simulink model "inverter"  (Simulink 8.4)
settings: Solver=ode23tb  StartTime=0.0  StopTime=0.1  MaxStep=.00001  RelTol=1e-3
libraries: powerlib x25, simulink x1
settings Model: Creator=jagadeeswari  LastModifiedBy=SELVA
settings SolverCC: InitialStep=0.0001

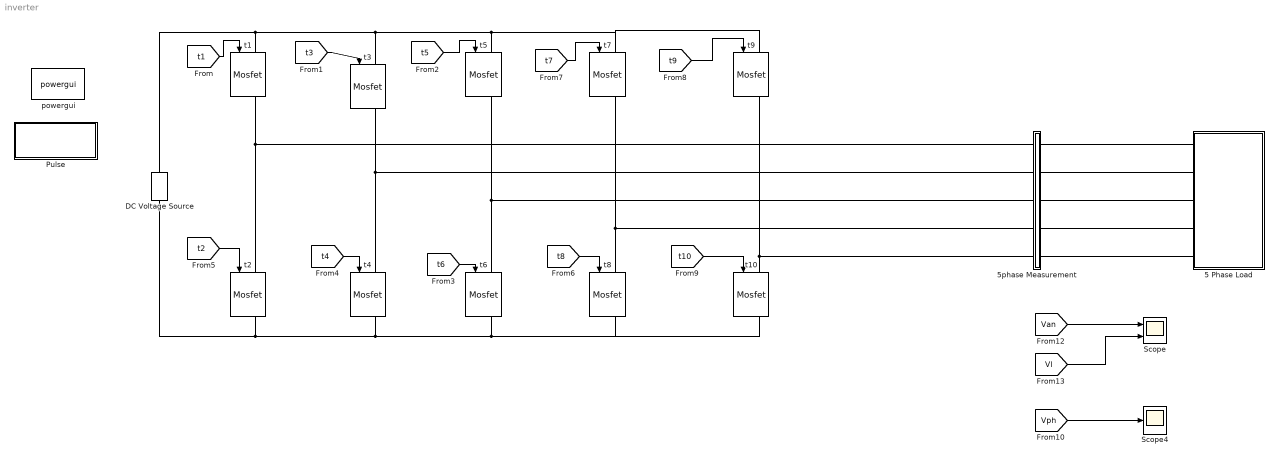
== system inverter ==
  5 Phase Load : Subsystem  mask{Vrms=70.7, f=50, P=1000}
      mask prompts: f "Frequency"; P "Active Power"
  5phase Measurement : Subsystem
  DC Voltage Source : powerlib/Electrical Sources/DC Voltage Source  Amplitude=100  Measurements=None
  Pulse : Subsystem
  Scope : Scope  NumInputPorts=2
      settings: YMin=-100~-60  YMax=100~80
  Scope4 : Scope
      settings: YMin=-100  YMax=100  SaveName=ScopeData4
  powergui : powerlib/powergui  Priority=1  SimulationMode=Continuous  SolverType=Tustin/Backward Euler (TBE)  SampleTime=50e-6  frequency=60  SPID=off  DisableSnubberDevices=off  DisableRonSwitches=off  DisableVfSwitches=off  SwTol=0  DisplayEquations=off  Interpol=off  methode=off  Ts=100  frequencyindice=0  Pbase=100e6  ErrMax=1e-4  Iterations=50  UnitsV=kV  UnitsW=MW  FunctionMessages=off  echomessages=off  HookPort=off  EnableUseOfTLC=off  x0status=blocks  RestoreLinks=warning  ResistiveCurrentMeasurement=off  Frange=[0:2:500]  Ylog=off  Xlog=on  ShowGrid=off  save=off  variable=ZData  structure=ScopeData4  ZoomFFT=off  StartTime=0.02  cycles=1  DisplayStyle=1  fundamental=50  FreqAxis=off  MaxFrequency=1000  frequencyindicesteady=1  RmsSteady=1  display=off
  t{1..10} (10 alike) : powerlib/Power Electronics/Mosfet  Ron=0.1  Lon=0  Rd=0.01  Vfd=0  IC=0  Rs=1e5  Cs=inf  Measurements=on
  wires:
  [t1] -> t1/1
  [t5] -> t5/1
  [t6] -> t6/1
  [t4] -> t4/1
  [t2] -> t2/1
  [t3] -> t3/1
  [t8] -> t8/1
  [t7] -> t7/1
  [t9] -> t9/1
  [t10] -> t10/1
  [Van] -> Scope/1
  [Vl] -> Scope/2
  [Vph] -> Scope4/1
  connections:
  DC Voltage Source/RConn1 -- t1/LConn1 -- t9/LConn1 -- t7/LConn1 -- t5/LConn1 -- t3/LConn1
  t2/RConn1 -- DC Voltage Source/LConn1 -- t4/RConn1 -- t10/RConn1 -- t8/RConn1 -- t6/RConn1
  t2/LConn1 -- 5phase Measurement/LConn1 -- t1/RConn1
  t7/RConn1 -- 5phase Measurement/LConn4 -- t8/LConn1
  t3/RConn1 -- t4/LConn1 -- 5phase Measurement/LConn2
  t6/LConn1 -- t5/RConn1 -- 5phase Measurement/LConn3
  t9/RConn1 -- 5phase Measurement/LConn5 -- t10/LConn1
  5 Phase Load/LConn1 -- 5phase Measurement/RConn1
  5phase Measurement/RConn2 -- 5 Phase Load/LConn2
  5 Phase Load/LConn3 -- 5phase Measurement/RConn3
  5phase Measurement/RConn4 -- 5 Phase Load/LConn4
  5 Phase Load/LConn5 -- 5phase Measurement/RConn5

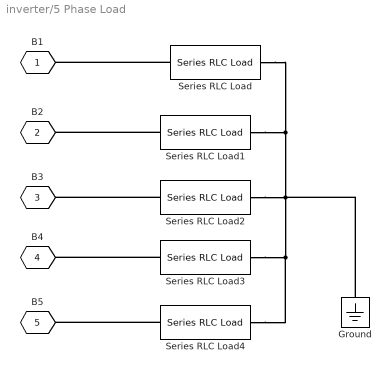
== system inverter/5 Phase Load ==
  Ground : powerlib/Elements/Ground  LConnTagsString=a
  Series RLC Load{,1..4} (5 alike) : powerlib/Elements/Series RLC Load  LConnTagsString=a  RConnTagsString=__new0  NominalVoltage=Vrms  NominalFrequency=f  ActivePower=P  InductivePower=0  CapacitivePower=0  Setx0=off  InitialVoltage=0  SetiL0=off  InitialCurrent=0  Measurements=None
  B1 : PMIOPort  Port=1  Side=Left
  B2 : PMIOPort  Port=2  Side=Left
  B3 : PMIOPort  Port=3  Side=Left
  B4 : PMIOPort  Port=4  Side=Left
  "B5 " : PMIOPort  Port=5  Side=Left
  connections:
  Series RLC Load/LConn1 -- B1/RConn1
  Series RLC Load1/LConn1 -- B2/RConn1
  Series RLC Load2/LConn1 -- B3/RConn1
  Series RLC Load3/LConn1 -- B4/RConn1
  Series RLC Load4/LConn1 -- "B5 "/RConn1
  Series RLC Load/RConn1 -- Series RLC Load1/RConn1 -- Series RLC Load2/RConn1 -- Ground/LConn1 -- Series RLC Load4/RConn1 -- Series RLC Load3/RConn1

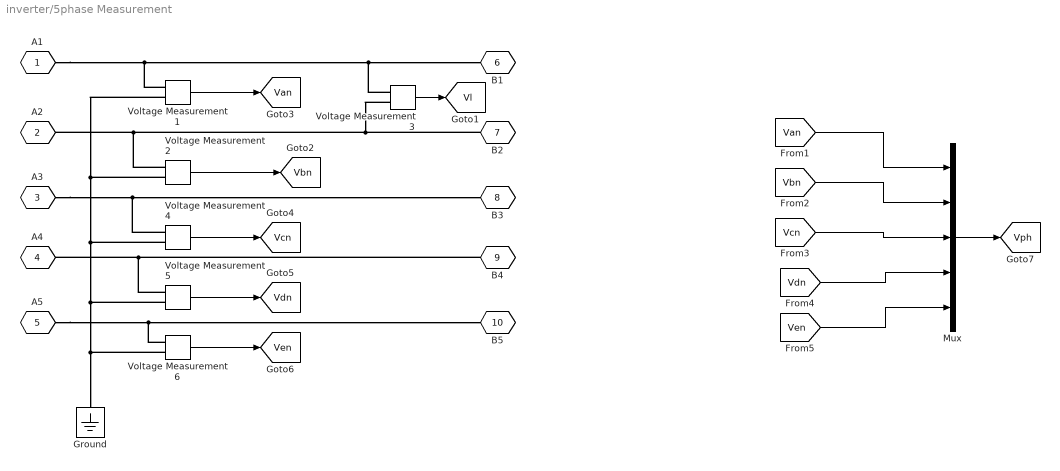
== system inverter/5phase Measurement ==
  Ground : powerlib/Elements/Ground  LConnTagsString=a
  Mux : Mux  Inputs=5
  Voltage Measurement{1..6} (6 alike) : powerlib/Measurements/Voltage Measurement  PhasorSimulation=off  OutputType=Complex  PSBequivalent=0
  A1 : PMIOPort  Port=1  Side=Right
  A2 : PMIOPort  Port=2  Side=Right
  A3 : PMIOPort  Port=3  Side=Right
  A4 : PMIOPort  Port=4  Side=Right
  A5 : PMIOPort  Port=5  Side=Right
  B1 : PMIOPort  Port=6  Side=Left
  B2 : PMIOPort  Port=7  Side=Left
  B3 : PMIOPort  Port=8  Side=Left
  B4 : PMIOPort  Port=9  Side=Left
  "B5 " : PMIOPort  Port=10  Side=Left
  tag scope: Van=global, Vbn=global, Vcn=global, Vdn=global, Ven=global, Vl=global, Vph=global
  wires:
  Voltage Measurement3/1 -> [Vl]
  Voltage Measurement2/1 -> [Vbn]
  Voltage Measurement1/1 -> [Van]
  Voltage Measurement6/1 -> [Ven]
  Voltage Measurement5/1 -> [Vdn]
  Voltage Measurement4/1 -> [Vcn]
  [Van] -> Mux/1
  [Vbn] -> Mux/2
  [Vcn] -> Mux/3
  [Vdn] -> Mux/4
  [Ven] -> Mux/5
  Mux/1 -> [Vph]
  connections:
  A1/RConn1 -- Voltage Measurement1/LConn1 -- Voltage Measurement3/LConn1 -- B1/RConn1
  B2/RConn1 -- Voltage Measurement2/LConn1 -- A2/RConn1 -- Voltage Measurement3/LConn2
  A3/RConn1 -- Voltage Measurement4/LConn1 -- B3/RConn1
  B4/RConn1 -- Voltage Measurement5/LConn1 -- A4/RConn1
  A5/RConn1 -- Voltage Measurement6/LConn1 -- "B5 "/RConn1
  Voltage Measurement1/LConn2 -- Voltage Measurement2/LConn2 -- Voltage Measurement4/LConn2 -- Voltage Measurement5/LConn2 -- Voltage Measurement6/LConn2 -- Ground/LConn1

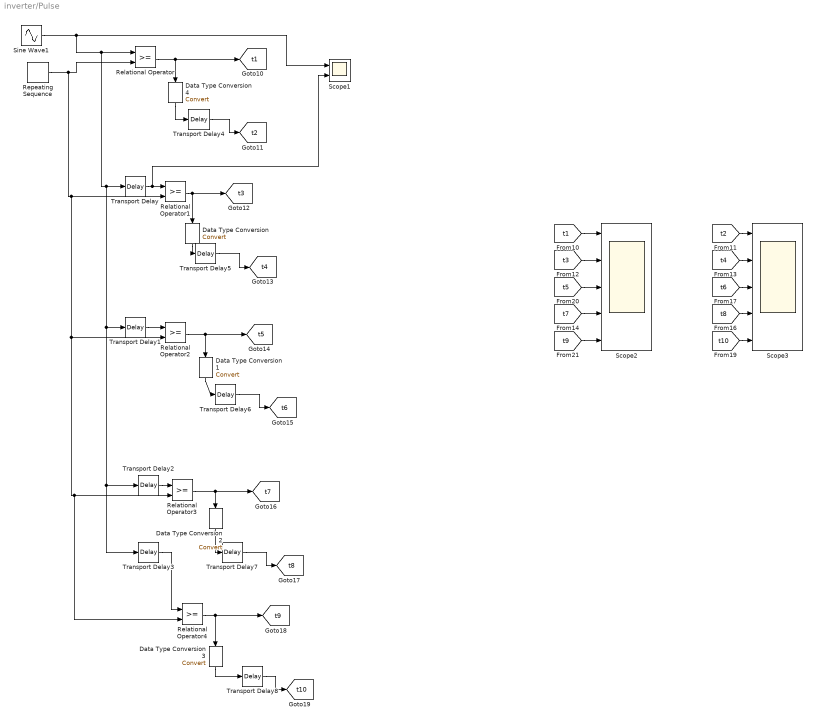
== system inverter/Pulse ==
  Data Type Conversion{,1..4} (5 alike) : DataTypeConversion
  Relational Operator{,1..4} (5 alike) : RelationalOperator  OutDataTypeStr=boolean
  Repeating Sequence : simulink/Sources/Repeating Sequence  rep_seq_t="[0  0.5*(1/1000)  1*(1/1000)]"  rep_seq_y=[0 1 0]
  Scope1 : Scope  NumInputPorts=2
      settings: YMin=-5~-5  YMax=5~5
  Scope2 : Scope  NumInputPorts=5
      settings: YMin=0~-5~-5~-5~-5  YMax=2~5~5~5~5  SaveName=ScopeData2
  Scope3 : Scope  NumInputPorts=5
      settings: YMin=-5~-5~-5~-5~-5  YMax=5~5~5~5~5  SaveName=ScopeData3
  Sine Wave1 : Sin  Frequency=2*pi*50  SampleTime=0
  Transport Delay : TransportDelay  DelayTime=(.01/180)*72
  Transport Delay1 : TransportDelay  DelayTime=(.01/180)*144
  Transport Delay2 : TransportDelay  DelayTime=(.01/180)*216
  Transport Delay3 : TransportDelay  DelayTime=(.01/180)*288
  Transport Delay{4..8} (5 alike) : TransportDelay  DelayTime=0.01
  tag scope: t10=global, t1=global, t2=global, t3=global, t4=global, t5=global, t6=global, t7=global, t8=global, t9=global
  wires:
  Transport Delay4/1 -> [t2]
  Sine Wave1/1 -> Scope1/1, Relational Operator/1, Transport Delay1/1, Transport Delay2/1, Transport Delay3/1, Transport Delay/1
  Repeating Sequence/1 -> Relational Operator4/2, Relational Operator3/2, Relational Operator2/2, Relational Operator1/2, Relational Operator/2
  Relational Operator/1 -> Data Type Conversion4/1, [t1]
  Transport Delay5/1 -> [t4]
  Relational Operator1/1 -> [t3], Data Type Conversion/1
  Transport Delay6/1 -> [t6]
  Relational Operator2/1 -> Data Type Conversion1/1, [t5]
  Transport Delay7/1 -> [t8]
  Relational Operator3/1 -> Data Type Conversion2/1, [t7]
  Transport Delay8/1 -> [t10]
  Relational Operator4/1 -> [t9], Data Type Conversion3/1
  Transport Delay1/1 -> Relational Operator2/1
  Transport Delay2/1 -> Relational Operator3/1
  Transport Delay3/1 -> Relational Operator4/1
  Transport Delay/1 -> Scope1/2, Relational Operator1/1
  Data Type Conversion/1 -> Transport Delay5/1
  Data Type Conversion1/1 -> Transport Delay6/1
  Data Type Conversion2/1 -> Transport Delay7/1
  Data Type Conversion3/1 -> Transport Delay8/1
  Data Type Conversion4/1 -> Transport Delay4/1
  [t1] -> Scope2/1
  [t10] -> Scope3/5
  [t3] -> Scope2/2
  [t5] -> Scope2/3
  [t7] -> Scope2/4
  [t9] -> Scope2/5
  [t8] -> Scope3/4
  [t6] -> Scope3/3
  [t2] -> Scope3/1
  [t4] -> Scope3/2
